simulink model "LQR"  (R2021a)
settings: Solver=ode45  StartTime=0.0  StopTime=t_final  MaxStep=params.maxStepSize  RelTol=1e-3
values from neighbouring files (symbols this model uses):
  K = lqr(A,B,C_z'*Q_dfl*C_z,R)    [LQRCtrl.m]
  maxW = 30    [LQRCtrl.m]
  params = Parameters()    [GenerateTrainigInput.m]    (also in LQRCtrl.m = Parameters(th_0); NewGenerateTrainigInput.m = NewParameters(5 , 5); NewModelValidation.m = NewParameters(); NewSysIdentification.m = NewParameters)
  z_d = [p_t;v_t; euler_t; omega_t; T_t; eta_t; gamma_t]    [LQRCtrl.m]
settings Model: Creator=Sopagna  LastModifiedBy=sarmiento
settings SolverCC: AlgebraicLoopSolver=LineSearch
settings DebuggingCC: SFMachineParentedDataDiag=warning

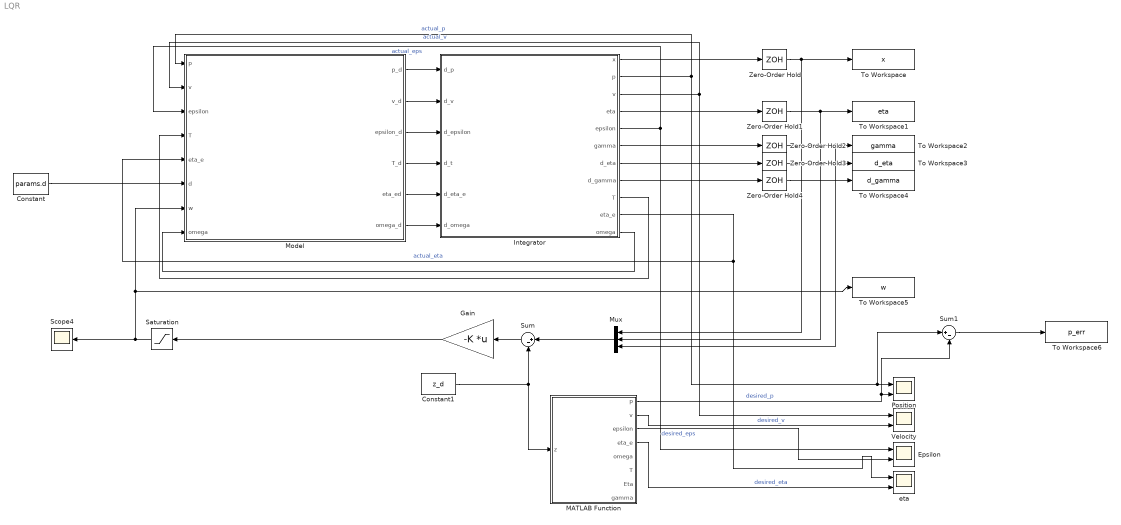
== system LQR ==
  Constant : Constant  Value=params.d
  Constant1 : Constant  Value=z_d
  Epsilon : Scope  NumInputPorts=2
  Gain : Gain  Gain=-K  Multiplication=Matrix(K*u) (u vector)
  Integrator : Subsystem
  MATLAB Function : MATLAB Function  TreatAsAtomicUnit=on
  Model : MATLAB Function  TreatAsAtomicUnit=on
  Mux : Mux  Inputs=3
  Position : Scope  NumInputPorts=2
  Saturation : Saturate  UpperLimit=maxW  LowerLimit=-maxW
  Scope4 : Scope
  Sum : Sum  Inputs=|+-
  Sum1 : Sum  Inputs=|+-
  To Workspace : ToWorkspace  VariableName=x  SampleTime=-1
      settings: Save2DSignal=2-D array (concatenate along first dimension)
  To Workspace1 : ToWorkspace  VariableName=eta  SampleTime=-1
      settings: Save2DSignal=2-D array (concatenate along first dimension)
  To Workspace2 : ToWorkspace  VariableName=gamma  SampleTime=-1
      settings: Save2DSignal=2-D array (concatenate along first dimension)
  To Workspace3 : ToWorkspace  VariableName=d_eta  SampleTime=-1
      settings: Save2DSignal=2-D array (concatenate along first dimension)
  To Workspace4 : ToWorkspace  VariableName=d_gamma  SampleTime=-1
      settings: Save2DSignal=2-D array (concatenate along first dimension)
  To Workspace5 : ToWorkspace  VariableName=w  SampleTime=-1
      settings: Save2DSignal=2-D array (concatenate along first dimension)
  To Workspace6 : ToWorkspace  VariableName=p_err  SampleTime=-1
      settings: Save2DSignal=2-D array (concatenate along first dimension)
  Velocity : Scope  NumInputPorts=2
  Zero-Order Hold{,1..4} (5 alike) : ZeroOrderHold  SampleTime=params.ST_id
  eta : Scope  NumInputPorts=2
  wires:
  Model/5(eta_ed) -> Integrator/5(d_eta_e)
  Constant/1 -> Model/6(d)
  Model/1(p_d) -> Integrator/1(d_p)
  Model/2(v_d) -> Integrator/2(d_v)
  Model/3(epsilon_d) -> Integrator/3(d_epsilon)
  Model/4(T_d) -> Integrator/4(d_t)
  Integrator/2(p) -> Model/1(p), Sum1/1, Position/1  "actual_p"
  Integrator/3(v) -> Model/2(v), Velocity/1  "actual_v"
  Integrator/5(epsilon) -> Model/3(epsilon), Epsilon/1  "actual_eps"
  Integrator/9(T) -> Model/4(T)
  Integrator/4(eta) -> Zero-Order Hold1/1
  Integrator/6(gamma) -> Zero-Order Hold2/1
  Integrator/7(d_eta) -> Zero-Order Hold3/1
  Integrator/8(d_gamma) -> Zero-Order Hold4/1
  Integrator/10(eta_e) -> eta/1, Model/5(eta_e)  "actual_eta"
  Zero-Order Hold/1 -> Mux/1, To Workspace/1
  Zero-Order Hold1/1 -> Mux/2, To Workspace1/1
  Zero-Order Hold2/1 -> Mux/3, To Workspace2/1
  Zero-Order Hold3/1 -> To Workspace3/1
  Zero-Order Hold4/1 -> To Workspace4/1
  Gain/1 -> Saturation/1
  Integrator/1(x) -> Zero-Order Hold/1
  Model/6(omega_d) -> Integrator/6(d_omega)
  Integrator/11(omega) -> Model/8(omega)
  Mux/1 -> Sum/1
  Sum/1 -> Gain/1
  Saturation/1 -> Scope4/1, Model/7(w), To Workspace5/1
  Constant1/1 -> MATLAB Function/1(z), Sum/2
  MATLAB Function/1(p) -> Sum1/2, Position/2  "desired_p"
  MATLAB Function/2(v) -> Velocity/2  "desired_v"
  MATLAB Function/3(epsilon) -> Epsilon/2  "desired_eps"
  MATLAB Function/4(eta_e) -> eta/2  "desired_eta"
  Sum1/1 -> To Workspace6/1

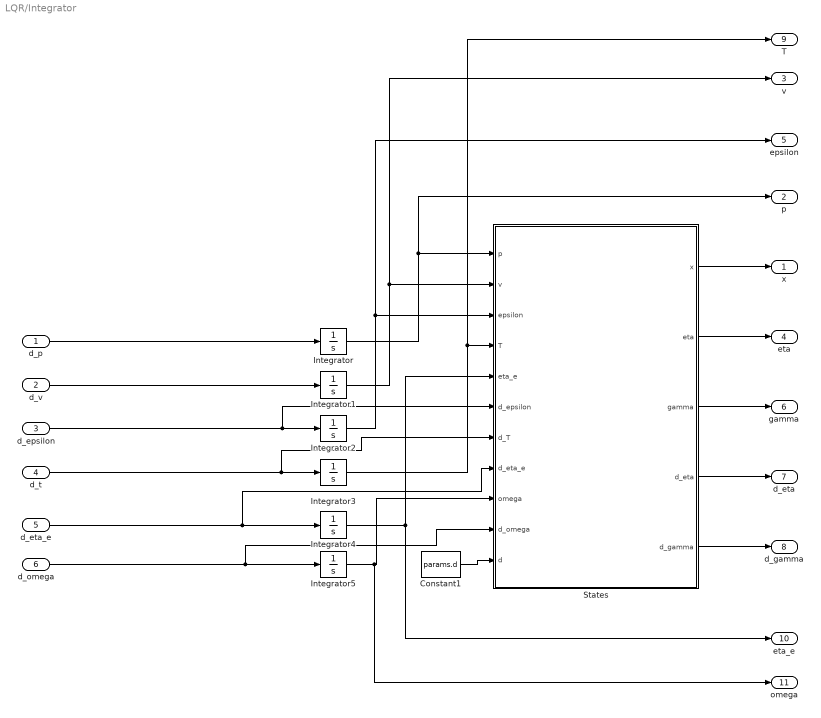
== system LQR/Integrator ==
  d_p : Inport
  d_v : Inport  Port=2
  d_epsilon : Inport  Port=3
  d_t : Inport  Port=4
  d_eta_e : Inport  Port=5
  d_omega : Inport  Port=6
  Constant1 : Constant  Value=params.d
  Integrator : Integrator  InitialCondition=params.p_0
  Integrator1 : Integrator  InitialCondition=params.v_0
  Integrator2 : Integrator  InitialCondition=params.epsilon_0
  Integrator3 : Integrator  InitialCondition=params.T_0
  Integrator4 : Integrator  InitialCondition=params.eta_e0
  Integrator5 : Integrator  InitialCondition=params.omega_0
  States : MATLAB Function  TreatAsAtomicUnit=on
  x : Outport
  p : Outport  Port=2
  v : Outport  Port=3
  eta : Outport  Port=4
  epsilon : Outport  Port=5
  gamma : Outport  Port=6
  d_eta : Outport  Port=7
  d_gamma : Outport  Port=8
  T : Outport  Port=9
  eta_e : Outport  Port=10
  omega : Outport  Port=11
  wires:
  d_eta_e/1 -> Integrator4/1, States/8(d_eta_e)
  d_epsilon/1 -> States/6(d_epsilon), Integrator2/1
  States/1(x) -> x/1
  d_p/1 -> Integrator/1
  States/2(eta) -> eta/1
  Integrator2/1 -> epsilon/1, States/3(epsilon)
  Integrator/1 -> p/1, States/1(p)
  Integrator1/1 -> v/1, States/2(v)
  d_t/1 -> States/7(d_T), Integrator3/1
  States/3(gamma) -> gamma/1
  Constant1/1 -> States/11(d)
  Integrator3/1 -> T/1, States/4(T)
  d_v/1 -> Integrator1/1
  States/5(d_gamma) -> d_gamma/1
  States/4(d_eta) -> d_eta/1
  Integrator4/1 -> eta_e/1, States/5(eta_e)
  d_omega/1 -> States/10(d_omega), Integrator5/1
  Integrator5/1 -> omega/1, States/9(omega)

== matlab function LQR/Integrator/States ==
  data: p input; v input; epsilon input; T input; eta_e input; d_epsilon input; d_T input; d_eta_e input; omega input; d_omega input; x output; eta output; gamma output; d_eta output; d_gamma output; d input
function [x,eta,gamma,d_eta,d_gamma] = fcn(p,v,epsilon,T,eta_e,d_epsilon,d_T,d_eta_e, omega, d_omega, d)
    %=================Original States=======================
    x = [p;v;epsilon; eta_e; omega;T]; 
    
    %=================Auxiliary variales====================
    eta = zeros(18,1);
    g = 9.81; %Gravity
    eta(1,:) = epsilon(1)*(epsilon(3)-d)*T;
    eta(2,:) = epsilon(2)*eta_e*T;
    eta(3,:) = epsilon(2)*(epsilon(3)-d)*T;
    eta(4,:) = epsilon(1)*eta_e*T;
    eta(5,:) = epsilon(1)^2*T;
    eta(6,:) = 2*epsilon(2)^2*T+g;

    eta(7,:) = ((epsilon(3) - d)*omega(2))/2;
    eta(8,:) = (epsilon(2)*omega(3))/2;
    eta(9,:) = (eta_e*omega(1))/2;
    eta(10,:) = (epsilon(1)*omega(3))/2;
    eta(11,:) = ((epsilon(3) - d)*omega(1))/2;
    eta(12,:) = (eta_e*omega(2))/2;
    eta(13,:) = (epsilon(2)*omega(1))/2;
    eta(14,:) = (epsilon(1)*omega(2))/2;
    eta(15,:) = (eta_e*omega(3))/2;
    eta(16,:) = (epsilon(1)*omega(1))/2;
    eta(17,:) = (epsilon(2)*omega(2))/2;
    eta(18,:) = ((epsilon(3) - d)*omega(3))/2;
    
    gamma = zeros(6,1);
    gamma(1,:) = epsilon(1)^2;
    gamma(2,:) = epsilon(2)^2;
    gamma(3,:) = (epsilon(3)-d)^2;
    gamma(4,:) = omega(1)^2;
    gamma(5,:) = omega(2)^2;
    gamma(6,:) = omega(3)^2;
%     gamma(7,:) = (eta_e)^2;
    %=============Time Derivative of Auxiliary Variables====================
    d_eta = zeros(18,1);

    d_eta(1,:)  =     T*d_epsilon(1)*(epsilon(3) - d) + T*d_epsilon(3)*epsilon(1) + d_T*epsilon(1)*(epsilon(3) - d);
    d_eta(2,:)  =     T*d_epsilon(2)*eta_e + epsilon(2)*d_eta_e*T + d_T*epsilon(2)*eta_e;
    d_eta(3,:)  =     T*d_epsilon(2)*(epsilon(3) - d) + T*d_epsilon(3)*epsilon(2) + d_T*epsilon(2)*(epsilon(3) - d);
    d_eta(4,:)  =     T*d_epsilon(1)*eta_e  + epsilon(1)*d_eta_e*T + d_T*epsilon(1)*eta_e;
    d_eta(5,:)  =     d_T*epsilon(1)^2 + 2*T*d_epsilon(1)*epsilon(1);
    d_eta(6,:)  =     2*d_T*epsilon(2)^2 + 4*T*d_epsilon(2)*epsilon(2);
    d_eta(7,:)  =     (d_omega(2)*(epsilon(3) - d))/2 + (d_epsilon(3)*omega(2))/2;
    d_eta(8,:)  =     (d_omega(3)*epsilon(2))/2 + (d_epsilon(2)*omega(3))/2;
    d_eta(9,:)  =     (d_omega(1)*eta_e)/2 + (d_eta_e*omega(1))/2;
    d_eta(10,:) =     (d_omega(3)*epsilon(1))/2 + (d_epsilon(1)*omega(3))/2;
    d_eta(11,:) =     (d_omega(1)*(epsilon(3) - d))/2 + (d_epsilon(3)*omega(1))/2;
    d_eta(12,:) =     (d_omega(2)*eta_e)/2 + (d_eta_e*omega(2))/2;
    d_eta(13,:) =     (d_omega(1)*epsilon(2))/2 + (d_epsilon(2)*omega(1))/2;
    d_eta(14,:) =     (d_omega(2)*epsilon(1))/2 + (d_epsilon(1)*omega(2))/2;
    d_eta(15,:) =     (d_omega(3)*eta_e)/2 + (d_eta_e*omega(3))/2;
    d_eta(16,:) =     (d_omega(1)*epsilon(1))/2 + (d_epsilon(1)*omega(1))/2;
    d_eta(17,:) =     (d_omega(2)*epsilon(2))/2 + (d_epsilon(2)*omega(2))/2;
    d_eta(18,:) =     (d_omega(3)*(epsilon(3) - d))/2 + (d_epsilon(3)*omega(3))/2;




    d_gamma = zeros(6,1);
    d_gamma(1,:) = 2*d_epsilon(1)*epsilon(1);
    d_gamma(2,:) = 2*d_epsilon(2)*epsilon(2);
    d_gamma(3,:) = 2*d_epsilon(3)*(epsilon(3) - d);
    d_gamma(4,:) = 2*d_omega(1)*omega(1);
    d_gamma(5,:) = 2*d_omega(2)*omega(2);
    d_gamma(6,:) = 2*d_omega(3)*omega(3);
%     d_gamma(7,:) = 2*d_eta_e*eta_e;

== matlab function LQR/Model ==
  data: p input size=[3 1]; v input size=[3 1]; epsilon input size=[3 1]; T input size=1; eta_e input size=1; d input size=1; w input size=[4 1]; p_d output size=[3 1]; v_d output size=[3 1]; epsilon_d output size=[3 1]; T_d output size=1; eta_ed output size=1; omega_d output; omega input
function [p_d,v_d,epsilon_d,T_d,eta_ed, omega_d] = fnc_training(p,v,epsilon,T,eta_e,d,w, omega)
% function [p_d,v_d,epsilon_d,T_d,eta_ed, omega_d] = fnc_training(p,v,epsilon,T,eta_e,d,w)
%==========================Input Variable================================
w1 = w(1:3); 
w2 = w(4); % Total Thrust
g = 9.81; % Gravity

%==========================Equation of Motion============================
p_d = v;    %Velocity
v_d = r_z(epsilon,eta_e,d)*T+[0;0;-g]; %Acceleration

%==========================First Way to get euler para derivative========
% epsilon_d = w1; %1st time derivative of euler parameters
% eta_e = sqrt(1-epsilon'*epsilon); % Angle of rotation

%==========================Second Way to get euler para derivative========
K =0.5;
euler = [epsilon;
        eta_e];
C = euler.'*euler-1;
J_E = J(euler);
% omega = 2*inv(J_E(1:3,:))*w1;
e_d = 0.5 *J_E* omega -K*C*euler;
epsilon_d = e_d(1:3);
eta_ed = e_d(4);
omega_d = w1;

T_d = w2; %Time derivative of total thrust

== matlab function LQR/MATLAB Function ==
  data: z input; p output; v output; epsilon output; eta_e output; omega output; T output; Eta output; gamma output
function [p, v, epsilon, eta_e, omega, T, Eta, gamma] = fcn(z)
p = z(1:3);
v = z(4:6);
epsilon = z(7:9);
eta_e = z(10);
omega = z(11:13);
T = z(14);
Eta = z(15:32);
gamma = z(33:38);
